simulink model "example_4_full_cascade"  (R2016a)
settings: Solver=VariableStepAuto  StartTime=0.0  StopTime=Tsim  MinStep=1e-5  RelTol=1e-3
values from neighbouring files (symbols this model uses):
  ref_A = 2.* [ 1.0, 1.0, 1.0, 1.0]    [init.m]
  ref_b = [ 0.0, 0.0, 0.0, 0.0]    [init.m]
  ref_p = [pi/2, 0.0, 0.0, 0.0]    [init.m]
  ref_w = 3.* [ 1.0, 0.0, 1.0, 0.0]    [init.m]
libraries: vrlib x4, simulink x1
settings Model: Creator=mgreiff  LastModifiedBy=mgreiff

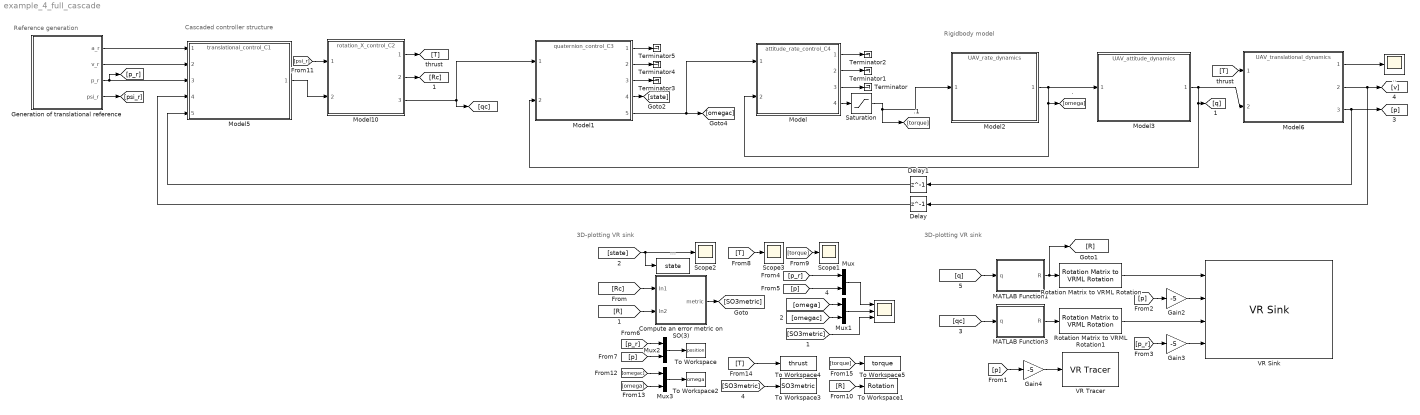
== system example_4_full_cascade ==
  note: 3D-plotting VR sink
  note: Rigidbody model
  note: Cascaded controller structure
  note: Reference generation
  note: 3D-plotting VR sink
  "                                     " : Scope  NumInputPorts=3
  .. : Scope
  ... : ToWorkspace  VariableName=state  SaveFormat=Timeseries  SampleTime=-1
  Compute an error metric on SO(3) : Subsystem
  Delay : Delay  DelayLength=1  InitialCondition=0  SampleTime=0.001
  Delay1 : Delay  DelayLength=1  InitialCondition=0  SampleTime=0.001
  Gain2 : Gain  Gain=-5
  Gain3 : Gain  Gain=-5
  Gain4 : Gain  Gain=-5
  Generation of translational reference : Subsystem
  MATLAB Function1 : MATLAB Function  TreatAsAtomicUnit=on
  MATLAB Function3 : MATLAB Function  TreatAsAtomicUnit=on
  Model : ModelReference  ModelNameDialog=attitude_rate_control_C4.slx  SimulationMode=Normal  ModelReferenceVersion=1.37
  Model1 : ModelReference  ModelNameDialog=quaternion_control_C3.slx  SimulationMode=Normal  ModelReferenceVersion=1.25
  Model10 : ModelReference  ModelNameDialog=rotation_X_control_C2.slx  SimulationMode=Normal  ModelReferenceVersion=1.129
  Model2 : ModelReference  ModelNameDialog=UAV_rate_dynamics.slx  SimulationMode=Normal  ModelReferenceVersion=1.9
  Model3 : ModelReference  ModelNameDialog=UAV_attitude_dynamics.slx  SimulationMode=Normal  ModelReferenceVersion=1.15
  Model5 : ModelReference  ModelNameDialog=translational_control_C1.slx  SimulationMode=Normal  ModelReferenceVersion=1.54
  Model6 : ModelReference  ModelNameDialog=UAV_translational_dynamics.slx  SimulationMode=Normal  ModelReferenceVersion=1.36
  Mux{,1..3} (4 alike) : Mux  Inputs=2
  Rotation Matrix to VRML Rotation : vrlib/Utilities/Rotation Matrix to VRML Rotation  maxzero=1e-12
  Rotation Matrix to VRML Rotation1 : vrlib/Utilities/Rotation Matrix to VRML Rotation  maxzero=1e-12
  Saturation : Saturate  UpperLimit=0.1  LowerLimit=-0.1
  Scope1 : Scope
  Scope2 : Scope
  Scope3 : Scope
  Terminator{,1..5} (6 alike) : Terminator
  To Workspace : ToWorkspace  VariableName=position  SaveFormat=Timeseries  SampleTime=-1
  To Workspace1 : ToWorkspace  VariableName=Rotation  SaveFormat=Timeseries  SampleTime=-1
  To Workspace2 : ToWorkspace  VariableName=omega  SaveFormat=Timeseries  SampleTime=-1
  To Workspace3 : ToWorkspace  VariableName=SO3metric  SaveFormat=Timeseries  SampleTime=-1
  To Workspace4 : ToWorkspace  VariableName=thrust  SaveFormat=Timeseries  SampleTime=-1
  To Workspace5 : ToWorkspace  VariableName=torque  SaveFormat=Timeseries  SampleTime=-1
  VR Sink : vrlib/VR Sink  InstantiateOnLoad=on  SampleTime=-1  ViewEnable=on  RemoteChange=off  RemoteView=off  FieldsWritten=body_axis.rotation.4.1.1.double#body_axis.translation.3.1.1.double#reference_axis.rotation.4.1.1.double#reference_axis.translation.3.1.1.double  WorldFileName=my_coordinate_systems.wrl  AutoView=on  VideoDimensions=[]  AllowVariableSize=off
  VR Tracer : vrlib/VR Tracer  VrmlFile=my_coordinate_systems.wrl  MarkerName=Sphere  UseLines=on  UseTriads=on  MarkerScale=[0.1,0.1,0.1]  MarkerColorSelection=Defined as RGB values  MarkerColor=red  rgbval=[0,0,1]  Ts=0.1  ForceViewerOpen=off  ConnectPlane=off  PlaneCoeff=[0 1 0 0]  ConnectPoint=None  PointCoord=[0 0 0]
  wires:
  [Rc] -> Compute an error metric on SO(3)/1(In1)
  [R] -> Compute an error metric on SO(3)/2(In2)
  Compute an error metric on SO(3)/1(metric) -> [SO3metric]
  [state] -> .../1, Scope2/1
  [SO3metric] -> "                                     "/3
  Mux/1 -> "                                     "/1
  Mux1/1 -> "                                     "/2
  [p] -> Mux/2
  [p_r] -> Mux/1
  [omega] -> Mux1/1
  [omegac] -> Mux1/2
  [qc] -> MATLAB Function3/1(q)
  [q] -> MATLAB Function1/1(q)
  [p] -> Gain2/1
  [p_r] -> Gain3/1
  Generation of translational reference/1(a_r) -> Model5/1
  Generation of translational reference/3("p_r ") -> [p_r], Model5/3
  Model6/3 -> Delay1/1, [p]
  Model6/2 -> Delay/1, [v]
  Model6/1 -> ../1
  Delay/1 -> Model5/4
  Delay1/1 -> Model5/5
  Model2/1 -> Model3/1, Model/2, [omega]
  [p] -> Gain4/1
  Gain4/1 -> VR Tracer/1
  Gain2/1 -> VR Sink/2
  Gain3/1 -> VR Sink/4
  Model1/4 -> [state]
  Model/3 -> Terminator/1
  Model/1 -> Terminator2/1
  Model/2 -> Terminator1/1
  Model1/1 -> Terminator5/1
  Model1/2 -> Terminator4/1
  Model1/3 -> Terminator3/1
  Rotation Matrix to VRML Rotation1/1 -> VR Sink/3
  Rotation Matrix to VRML Rotation/1 -> VR Sink/1
  MATLAB Function1/1(R) -> [R], Rotation Matrix to VRML Rotation/1
  MATLAB Function3/1(R) -> Rotation Matrix to VRML Rotation1/1
  Model/4 -> Saturation/1
  [p] -> Mux2/2
  [p_r] -> Mux2/1
  Mux2/1 -> To Workspace/1
  Generation of translational reference/2(v_r) -> Model5/2
  Model10/3 -> [qc], Model1/1
  Model5/1 -> Model10/2
  [T] -> Model6/1
  Model10/1 -> [T]
  Model10/2 -> [Rc]
  Generation of translational reference/4(psi_r) -> [psi_r]
  [T] -> Scope3/1
  Model3/1 -> Model1/2, [q], Model6/2
  [torque] -> Scope1/1
  [R] -> To Workspace1/1
  [psi_r] -> Model10/1
  Model1/5 -> Model/1, [omegac]
  Saturation/1 -> [torque], Model2/1
  [omega] -> Mux3/2
  [omegac] -> Mux3/1
  Mux3/1 -> To Workspace2/1
  [SO3metric] -> To Workspace3/1
  [T] -> To Workspace4/1
  [torque] -> To Workspace5/1

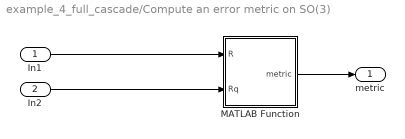
== system example_4_full_cascade/Compute an error metric on SO(3) ==
  In1 : Inport
  In2 : Inport  Port=2
  MATLAB Function : MATLAB Function  TreatAsAtomicUnit=on
  metric : Outport
  wires:
  MATLAB Function/1(metric) -> metric/1
  In1/1 -> MATLAB Function/1(R)
  In2/1 -> MATLAB Function/2(Rq)

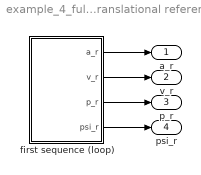
== system example_4_full_cascade/Generation of translational reference ==
  first sequence (loop) : Subsystem
  a_r : Outport  PortDimensions=3
  v_r : Outport  Port=2  PortDimensions=3
  "p_r " : Outport  Port=3  PortDimensions=3
  psi_r : Outport  Port=4  PortDimensions=1
  wires:
  first sequence (loop)/3("p_r ") -> "p_r "/1
  first sequence (loop)/4(psi_r) -> psi_r/1
  first sequence (loop)/1(a_r) -> a_r/1
  first sequence (loop)/2(v_r) -> v_r/1

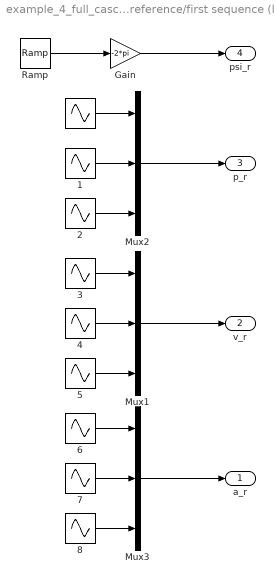
== system example_4_full_cascade/Generation of translational reference/first sequence (loop) ==
  " " : Sin  Amplitude=ref_A(1)  Bias=ref_b(1)  Frequency=ref_w(1)  Phase=ref_p(1)
  " 1" : Sin  Amplitude=ref_A(2)  Bias=ref_b(2)  Frequency=ref_w(2)  Phase=ref_p(2)
  " 2" : Sin  Amplitude=ref_A(3)  Bias=ref_b(3)  Frequency=ref_w(3)  Phase=ref_p(3)
  " 3" : Sin  Amplitude=ref_A(1)*ref_w(1)  Bias=ref_b(1)  Frequency=ref_w(1)  Phase=ref_p(1)+pi/2
  " 4" : Sin  Amplitude=ref_A(2)*ref_w(2)  Bias=ref_b(2)  Frequency=ref_w(2)  Phase=ref_p(2)+pi/2
  " 5" : Sin  Amplitude=ref_A(3)*ref_w(3)  Bias=ref_b(3)  Frequency=ref_w(3)  Phase=ref_p(3)+pi/2
  " 6" : Sin  Amplitude=ref_A(1)*ref_w(1)*ref_w(1)  Bias=ref_b(1)  Frequency=ref_w(1)  Phase=ref_p(1)-pi
  " 7" : Sin  Amplitude=ref_A(2)*ref_w(2)*ref_w(2)  Bias=ref_b(2)  Frequency=ref_w(2)  Phase=ref_p(2)-pi
  " 8" : Sin  Amplitude=ref_A(3)*ref_w(3)*ref_w(3)  Bias=ref_b(3)  Frequency=ref_w(3)  Phase=ref_p(3)-pi
  Gain : Gain  Gain=-2*pi
  Mux1 : Mux  Inputs=3
  Mux2 : Mux  Inputs=3
  Mux3 : Mux  Inputs=3
  Ramp : simulink/Sources/Ramp  slope=1  start=0  X0=0
  a_r : Outport  PortDimensions=3
  v_r : Outport  Port=2  PortDimensions=3
  "p_r " : Outport  Port=3  PortDimensions=3
  psi_r : Outport  Port=4  PortDimensions=1
  wires:
  " 5"/1 -> Mux1/3
  Mux1/1 -> v_r/1
  Gain/1 -> psi_r/1
  Mux3/1 -> a_r/1
  " 3"/1 -> Mux1/1
  Mux2/1 -> "p_r "/1
  " 4"/1 -> Mux1/2
  " 1"/1 -> Mux2/2
  " 7"/1 -> Mux3/2
  " 8"/1 -> Mux3/3
  " "/1 -> Mux2/1
  Ramp/1 -> Gain/1
  " 2"/1 -> Mux2/3
  " 6"/1 -> Mux3/1

== matlab function example_4_full_cascade/Compute an error metric on SO(3)/MATLAB Function ==
  data: R input; metric output; Rq input
function metric = fcn(R, Rq)
%#codegen
metric = 0.5.*trace(eye(3) - Rq'*R);
end

== matlab function example_4_full_cascade/MATLAB Function1 ==
  data: q input; R output
function R = fcn(q)
q = q./norm(q);
qw = q(1);
qx = q(2);
qy = q(3);
qz = q(4);

R = [qw^2 + qx^2-qy^2-qz^2, 2*(qx*qy-qw*qz)    , 2*(qx*qz+qw*qy);
     2*(qx*qy+qw*qz)    , qw^2-qx^2+qy^2-qz^2, 2*(qy*qz-qw*qx);
     2*(qx*qz-qw*qy)    , 2*(qy*qz+qw*qx)    , qw^2-qx^2-qy^2+qz^2];

== matlab function example_4_full_cascade/MATLAB Function3 ==
  data: q input; R output
function R = fcn(q)
q = q./norm(q);
qw = q(1);
qx = q(2);
qy = q(3);
qz = q(4);

R = [qw^2 + qx^2-qy^2-qz^2, 2*(qx*qy-qw*qz)    , 2*(qx*qz+qw*qy);
     2*(qx*qy+qw*qz)    , qw^2-qx^2+qy^2-qz^2, 2*(qy*qz-qw*qx);
     2*(qx*qz-qw*qy)    , 2*(qy*qz+qw*qx)    , qw^2-qx^2-qy^2+qz^2];
